simulink model "sim_hinf_bike"  (R2022a)
settings: Solver=VariableStepAuto  StartTime=0.0  StopTime=10.0  RelTol=1e-3
settings Model: Creator=Jonas  LastModifiedBy=Jonas

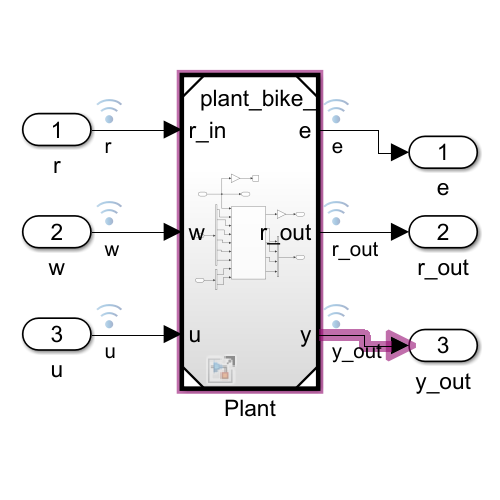
[thumbnail: Simulink's stored preview of the top-level diagram]
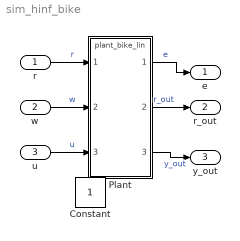
== system sim_hinf_bike ==
  r : Inport
  w : Inport  Port=2
  u : Inport  Port=3
  Plant : ModelReference  ModelNameDialog=plant_bike_lin  SimulationMode=Normal  ModelReferenceVersion=1.11
  e : Outport
  r_out : Outport  Port=2
  y_out : Outport  Port=3
  Constant : Constant  IOType=siggen
  wires:
  Plant/1 -> e/1  "e"
  u/1 -> Plant/3  "u"
  r/1 -> Plant/1  "r"
  w/1 -> Plant/2  "w"
  Plant/2 -> r_out/1  "r_out"
  Plant/3 -> y_out/1  "y_out"
